simulink model "sim"  (R2018a)
settings: Solver=VariableStepAuto  StartTime=0.0  StopTime=100  RelTol=1e-3
libraries: fuzblock x1
settings Model: Creator=daniel  LastModifiedBy=daniel

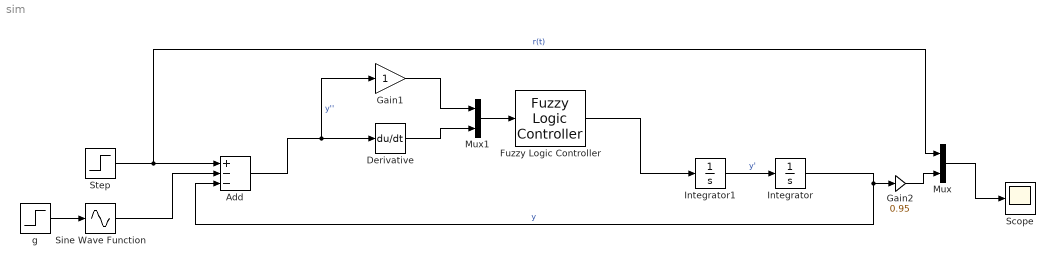
== system sim ==
  Add : Sum  Inputs=+--
  Derivative : Derivative
  Fuzzy Logic Controller : fuzblock/Fuzzy Logic  Controller  FIS=sys  OutputSampleNumber=101  DataType=double  FuzzifiedInputs=off  RuleFiringStrengths=off  RuleOutputs=off  AggregatedOutputs=off  SimulateUsing=Interpreted execution  OutOfRangeInputValueMessage=warning  NoRuleFiredMessage=warning  EmptyOutputFuzzySetMessage=warning
  Gain1 : Gain
  Gain2 : Gain  Gain=0.95
  Integrator : Integrator
  Integrator1 : Integrator
  Mux : Mux  Inputs=2
  Mux1 : Mux  Inputs=2
  Scope : Scope
  Sine Wave Function : Sin  TimeSource=Use external signal  SampleTime=0
  Step : Step  Time=0  SampleTime=0
  g : Step  Time=0  After=9.8  SampleTime=0
  wires:
  Step/1 -> Add/1, Mux/1  "r(t)"
  Mux/1 -> Scope/1
  g/1 -> Sine Wave Function/1
  Sine Wave Function/1 -> Add/2
  Add/1 -> Gain1/1, Derivative/1  "y''"
  Integrator1/1 -> Integrator/1  "y'"
  Integrator/1 -> Add/3, Gain2/1  "y"
  Mux1/1 -> Fuzzy Logic Controller/1
  Gain1/1 -> Mux1/1
  Derivative/1 -> Mux1/2
  Fuzzy Logic Controller/1 -> Integrator1/1
  Gain2/1 -> Mux/2
